simulink model "atrias_system_testing_delay"  (R2014a)
settings: Solver=FixedStepDiscrete  StartTime=0.0  StopTime=inf  FixedStep=sample_time  RelTol=1e-3
PreLoadFcn:
  | set_sampletime
PostLoadFcn:
  | set_sampletime
InitFcn:
  | sys_params
StartFcn:
  | set_sampletime
values from neighbouring files (symbols this model uses):
  A_lpf_velocity = 1 + B1_lpf_velocity + B2_lpf_velocity    [daq_params_osu.m]
  B1_lpf_velocity = -2*exp(-lpf_damping*fcut_velocity*sample_time)*cos(fcut_velocity*sample_time*sqrt(1-lpf_damping^2))    [daq_params_osu.m]
  B2_lpf_velocity = exp(-2*lpf_damping*fcut_velocity*sample_time)    [daq_params_osu.m]
  BOOM_MAX_ENCODER_TICKS = 2^17 - 1    (= 131071)    [daq_params_osu.m]
  BOOM_PITCH_CAL_VALUE_RAD = 0    [daq_params_osu.m]
  BOOM_PITCH_CAL_VALUE_TICKS = 43809    [daq_params_osu.m]
  BOOM_PITCH_ENCODER_RAD_PER_TICK = -2*pi / (2^17 * 2)    (= -2.39684498107e-05)    [daq_params_osu.m]
  BOOM_ROLL_CAL_VALUE_RAD = 0.1271    [daq_params_osu.m]
  BOOM_ROLL_CAL_VALUE_TICKS = 9318    [daq_params_osu.m]
  BOOM_ROLL_ENCODER_RAD_PER_TICK = 2*pi / (2^17 * 7)    (= 6.84812851735e-06)    [daq_params_osu.m]
  BOOM_YAW_ENCODER_RAD_PER_TICK = 2*pi / (2^17 * 9.6)    (= 4.9934270439e-06)    [daq_params_osu.m]
  CURRENT_LIMIT = 100    [daq_params_osu.m]
  fcut_smooth = 16*(2*pi)    (= 100.530964915)    [daq_params_osu.m]
  fcut_unwrap = 8*(2*pi)    (= 50.2654824574)    [daq_params_osu.m]
  gui_disable_cmd = 0    [daq_params_osu.m]
  gui_enable_cmd = 0    [daq_params_osu.m]
  gui_estop_cmd = 0    [daq_params_osu.m]
  gui_reset_cmd = 0    [daq_params_osu.m]
  HIP_ABS_ENCODER_RAD_PER_TICK = 2*pi / 2^13    (= 0.000766990393943)    [daq_params_osu.m]
  HIP_ABS_MAX_ENCODER_TICKS = 2^13 - 1    (= 8191)    [daq_params_osu.m]
  HIP_INC_ENCODER_RAD_PER_TICK = 2*pi / (2500 * 4 * 57)    (= 1.10231321179e-05)    [daq_params_osu.m]
  HIP_INC_MAX_ENCODER_TICKS = 2^16 - 1    (= 65535)    [daq_params_osu.m]
  HIP_MOTOR_CONSTANT = 0.184    [daq_params_osu.m]
  HIP_MTR_GEAR_RATIO = 57    [daq_params_osu.m]
  HIP_MTR_MAX_TORQUE = MTR_HIP_MAX_CURRENT*HIP_MOTOR_CONSTANT*HIP_MTR_GEAR_RATIO    (= 629.28)    [daq_params_osu.m]
  INC_ENC_DIRS = -[ LEG1_MOTOR_A_DIRECTION ... (first row only)    [daq_params_osu.m]
  INC_ENC_RAD_PER_TICK = 2*pi/14000/LEG_MTR_GEAR_RATIO    (= 8.97597901026e-06)    [daq_params_osu.m]
  k_sea = 4118    [sys_params.m]
  LEFT_HIP_CALIB_POS = 0    [daq_params_osu.m]
  LEFT_HIP_CALIB_VAL = 7192 - 2^13    (= -1000)    [daq_params_osu.m]
  LEFT_MOTOR_HIP_DIRECTION = -1.0    (= -1)    [daq_params_osu.m]
  LEG1_LEG_A_CALIB_VAL = 265417675    [daq_params_osu.m]
  LEG1_LEG_A_RAD_PER_CNT = -9.8039216e-09    [daq_params_osu.m]
  LEG1_LEG_B_CALIB_VAL = 175319150    [daq_params_osu.m]
  LEG1_LEG_B_RAD_PER_CNT = -9.8039216e-09    [daq_params_osu.m]
  LEG1_MOTOR_A_DIRECTION = -1.0    (= -1)    [daq_params_osu.m]
  LEG1_MOTOR_B_DIRECTION = -1.0    (= -1)    [daq_params_osu.m]
  LEG1_TRAN_A_CALIB_VAL = 143046540    [daq_params_osu.m]
  LEG1_TRAN_A_RAD_PER_CNT = 9.8039216e-09    [daq_params_osu.m]
  LEG1_TRAN_B_CALIB_VAL = 142356572    [daq_params_osu.m]
  LEG1_TRAN_B_RAD_PER_CNT = -9.8039216e-09    [daq_params_osu.m]
  LEG2_LEG_A_CALIB_VAL = 264357825    [daq_params_osu.m]
  LEG2_LEG_A_RAD_PER_CNT = -9.8039216e-09    [daq_params_osu.m]
  LEG2_LEG_B_CALIB_VAL = 261444054    [daq_params_osu.m]
  LEG2_LEG_B_RAD_PER_CNT = 9.8039216e-09    [daq_params_osu.m]
  LEG2_MOTOR_A_DIRECTION = 1.0    (= 1)    [daq_params_osu.m]
  LEG2_MOTOR_B_DIRECTION = 1.0    (= 1)    [daq_params_osu.m]
  LEG2_TRAN_A_CALIB_VAL = 142300933    [daq_params_osu.m]
  LEG2_TRAN_A_RAD_PER_CNT = 9.8039216e-09    [daq_params_osu.m]
  LEG2_TRAN_B_CALIB_VAL = 142287413    [daq_params_osu.m]
  LEG2_TRAN_B_RAD_PER_CNT = -9.8039216e-09    [daq_params_osu.m]
  LEG_A_CALIB_LOC = pi + 0.305432619099008    (= 3.44702527269)    [daq_params_osu.m]
  LEG_B_CALIB_LOC = pi - 0.305432619099008    (= 2.83616003449)    [daq_params_osu.m]
  LEG_MOTOR_CONSTANT = 0.119    [daq_params_osu.m]
  LEG_MTR_GEAR_RATIO = 50    [daq_params_osu.m]
  LEG_MTR_MAX_TORQUE = MTR_MAX_CURRENT*LEG_MOTOR_CONSTANT*LEG_MTR_GEAR_RATIO    (= 922.25)    [daq_params_osu.m]
  max_encoder_velocity = 200    [daq_params_osu.m]
  MEDULLA_ADC_MAX_VOLTS = 2.70    (= 2.7)    [daq_params_osu.m]
  MEDULLA_ADC_OFFSET_COUNTS = 172    [daq_params_osu.m]
  MEDULLA_STATE_ERROR = 5    [daq_params_osu.m]
  MEDULLA_STATE_HALT = 4    [daq_params_osu.m]
  MEDULLA_STATE_IDLE = 0    [daq_params_osu.m]
  MEDULLA_STATE_RESET = 6    [daq_params_osu.m]
  MEDULLA_STATE_RUN = 2    [daq_params_osu.m]
  MEDULLA_TIMER_FREQ = 32e6    (= 32000000)    [daq_params_osu.m]
  MOTOR_POSITION_LIMITS_LOWER = [2.5; 1.4; 0.4]    [daq_params_osu.m]
  MOTOR_POSITION_LIMITS_UPPER = [4.9; 3.8; 2.5]    [daq_params_osu.m]
  MTR_HIP_MAX_CURRENT = 60.0    (= 60)    [daq_params_osu.m]
  MTR_MAX_CONT_CURRENT = 100.0    (= 100)    [daq_params_osu.m]
  MTR_MAX_COUNT = 19900    [daq_params_osu.m]
  MTR_MAX_CURRENT = 155.0    (= 155)    [daq_params_osu.m]
  nom_sample_time = 0.001    [sys_params.m]
  RIGHT_HIP_CALIB_POS = 0    [daq_params_osu.m]
  RIGHT_HIP_CALIB_VAL = 1091    [daq_params_osu.m]
  RIGHT_MOTOR_HIP_DIRECTION = 1.0    (= 1)    [daq_params_osu.m]
  sample_time = 1/update_freq    (= 0.001)    [daq_params_osu.m]
  sensor_start_time = 8    [daq_params_osu.m]
undefined symbols (not defined in the file or in its folder): max_sensor_velocity
libraries: xpcethercatlib x196, simulink x50, slrtlib x4, dspswit3 x1
(part 4 of 4)

== system atrias_system_testing_delay/DAQ/Elmo Back Right/Drive state transition ==
  Status : Inport
  Bitwise Operator : simulink/Logic and Bit Operations/Bitwise Operator  logicop=AND  UseBitMask=on  BitMask=hex2dec('ff')  BitMaskRealWorld=Stored Integer
  Bitwise Operator1 : simulink/Logic and Bit Operations/Bitwise Operator  logicop=AND  UseBitMask=on  BitMask=hex2dec('80')  BitMaskRealWorld=Stored Integer
  Compare To Constant : simulink/Logic and Bit Operations/Compare To Constant  relop===  const=80  OutDataTypeStr=boolean
  Compare To Constant1 : simulink/Logic and Bit Operations/Compare To Constant  relop===  const=49  OutDataTypeStr=boolean
  Compare To Constant2 : simulink/Logic and Bit Operations/Compare To Constant  relop===  const=51  OutDataTypeStr=boolean
  Compare To Constant3 : simulink/Logic and Bit Operations/Compare To Constant  relop===  const=55  OutDataTypeStr=boolean
  Compare To Zero : simulink/Logic and Bit Operations/Compare To Zero  relop=~=  OutDataTypeStr=boolean
  Constant : Constant  Value=0  OutDataTypeStr=uint16
  Constant1 : Constant  Value=128  OutDataTypeStr=uint16
  Constant2 : Constant  Value=6  OutDataTypeStr=uint16
  Constant3 : Constant  Value=7  OutDataTypeStr=uint16
  Constant4 : Constant  Value=15  OutDataTypeStr=uint16
  Constant5 : Constant  Value=15  OutDataTypeStr=uint16
  Switch{,1..4} (5 alike) : Switch  Criteria=u2 > Threshold
  Control : Outport
  wires:
  Status/1 -> Bitwise Operator/1, Bitwise Operator1/1
  Bitwise Operator1/1 -> Compare To Zero/1
  Compare To Zero/1 -> Switch/2
  Constant1/1 -> Switch/1
  Constant/1 -> Switch/3
  Compare To Constant/1 -> Switch1/2
  Switch/1 -> Switch1/3
  Bitwise Operator/1 -> Compare To Constant3/1, Compare To Constant2/1, Compare To Constant1/1, Compare To Constant/1
  Constant2/1 -> Switch1/1
  Compare To Constant1/1 -> Switch2/2
  Switch1/1 -> Switch2/3
  Constant3/1 -> Switch2/1
  Compare To Constant2/1 -> Switch3/2
  Switch2/1 -> Switch3/3
  Constant4/1 -> Switch3/1
  Compare To Constant3/1 -> Switch4/2
  Switch3/1 -> Switch4/3
  Constant5/1 -> Switch4/1
  Switch4/1 -> Control/1

== system atrias_system_testing_delay/DAQ/Elmo Front Left/Drive state transition ==
  Status : Inport
  Bitwise Operator : simulink/Logic and Bit Operations/Bitwise Operator  logicop=AND  UseBitMask=on  BitMask=hex2dec('ff')  BitMaskRealWorld=Stored Integer
  Bitwise Operator1 : simulink/Logic and Bit Operations/Bitwise Operator  logicop=AND  UseBitMask=on  BitMask=hex2dec('80')  BitMaskRealWorld=Stored Integer
  Compare To Constant : simulink/Logic and Bit Operations/Compare To Constant  relop===  const=80  OutDataTypeStr=boolean
  Compare To Constant1 : simulink/Logic and Bit Operations/Compare To Constant  relop===  const=49  OutDataTypeStr=boolean
  Compare To Constant2 : simulink/Logic and Bit Operations/Compare To Constant  relop===  const=51  OutDataTypeStr=boolean
  Compare To Constant3 : simulink/Logic and Bit Operations/Compare To Constant  relop===  const=55  OutDataTypeStr=boolean
  Compare To Zero : simulink/Logic and Bit Operations/Compare To Zero  relop=~=  OutDataTypeStr=boolean
  Constant : Constant  Value=0  OutDataTypeStr=uint16
  Constant1 : Constant  Value=128  OutDataTypeStr=uint16
  Constant2 : Constant  Value=6  OutDataTypeStr=uint16
  Constant3 : Constant  Value=7  OutDataTypeStr=uint16
  Constant4 : Constant  Value=15  OutDataTypeStr=uint16
  Constant5 : Constant  Value=15  OutDataTypeStr=uint16
  Switch{,1..4} (5 alike) : Switch  Criteria=u2 > Threshold
  Control : Outport
  wires:
  Status/1 -> Bitwise Operator/1, Bitwise Operator1/1
  Bitwise Operator1/1 -> Compare To Zero/1
  Compare To Zero/1 -> Switch/2
  Constant1/1 -> Switch/1
  Constant/1 -> Switch/3
  Compare To Constant/1 -> Switch1/2
  Switch/1 -> Switch1/3
  Bitwise Operator/1 -> Compare To Constant3/1, Compare To Constant2/1, Compare To Constant1/1, Compare To Constant/1
  Constant2/1 -> Switch1/1
  Compare To Constant1/1 -> Switch2/2
  Switch1/1 -> Switch2/3
  Constant3/1 -> Switch2/1
  Compare To Constant2/1 -> Switch3/2
  Switch2/1 -> Switch3/3
  Constant4/1 -> Switch3/1
  Compare To Constant3/1 -> Switch4/2
  Switch3/1 -> Switch4/3
  Constant5/1 -> Switch4/1
  Switch4/1 -> Control/1

== system atrias_system_testing_delay/DAQ/Elmo Front Right/Drive state transition ==
  Status : Inport
  Bitwise Operator : simulink/Logic and Bit Operations/Bitwise Operator  logicop=AND  UseBitMask=on  BitMask=hex2dec('ff')  BitMaskRealWorld=Stored Integer
  Bitwise Operator1 : simulink/Logic and Bit Operations/Bitwise Operator  logicop=AND  UseBitMask=on  BitMask=hex2dec('80')  BitMaskRealWorld=Stored Integer
  Compare To Constant : simulink/Logic and Bit Operations/Compare To Constant  relop===  const=80  OutDataTypeStr=boolean
  Compare To Constant1 : simulink/Logic and Bit Operations/Compare To Constant  relop===  const=49  OutDataTypeStr=boolean
  Compare To Constant2 : simulink/Logic and Bit Operations/Compare To Constant  relop===  const=51  OutDataTypeStr=boolean
  Compare To Constant3 : simulink/Logic and Bit Operations/Compare To Constant  relop===  const=55  OutDataTypeStr=boolean
  Compare To Zero : simulink/Logic and Bit Operations/Compare To Zero  relop=~=  OutDataTypeStr=boolean
  Constant : Constant  Value=0  OutDataTypeStr=uint16
  Constant1 : Constant  Value=128  OutDataTypeStr=uint16
  Constant2 : Constant  Value=6  OutDataTypeStr=uint16
  Constant3 : Constant  Value=7  OutDataTypeStr=uint16
  Constant4 : Constant  Value=15  OutDataTypeStr=uint16
  Constant5 : Constant  Value=15  OutDataTypeStr=uint16
  Switch{,1..4} (5 alike) : Switch  Criteria=u2 > Threshold
  Control : Outport
  wires:
  Status/1 -> Bitwise Operator/1, Bitwise Operator1/1
  Bitwise Operator1/1 -> Compare To Zero/1
  Compare To Zero/1 -> Switch/2
  Constant1/1 -> Switch/1
  Constant/1 -> Switch/3
  Compare To Constant/1 -> Switch1/2
  Switch/1 -> Switch1/3
  Bitwise Operator/1 -> Compare To Constant3/1, Compare To Constant2/1, Compare To Constant1/1, Compare To Constant/1
  Constant2/1 -> Switch1/1
  Compare To Constant1/1 -> Switch2/2
  Switch1/1 -> Switch2/3
  Constant3/1 -> Switch2/1
  Compare To Constant2/1 -> Switch3/2
  Switch2/1 -> Switch3/3
  Constant4/1 -> Switch3/1
  Compare To Constant3/1 -> Switch4/2
  Switch3/1 -> Switch4/3
  Constant5/1 -> Switch4/1
  Switch4/1 -> Control/1

== system atrias_system_testing_delay/DAQ/calibrate_and_convert_to_rad/calibrate_abs_encoder ==
  encoder_ticks : Inport
  cal_pt_ticks : Inport  Port=2
  cal_pt_rad : Inport  Port=3
  ticks_to_rad_const : Inport  Port=4
  Product : Product  RndMeth=Zero
  Sum : Sum  Inputs=|+-
  Sum1 : Sum  Inputs=|++
  angle [rad] : Outport
  wires:
  Sum/1 -> Product/1  "tick_diff"
  encoder_ticks/1 -> Sum/1  "encoder_ticks"
  Product/1 -> Sum1/1  "rad_diff"
  ticks_to_rad_const/1 -> Product/2  "ticks_to_rad_const"
  cal_pt_ticks/1 -> Sum/2  "calibration_point_ticks"
  Sum1/1 -> angle [rad]/1  "calibrated_angle"
  cal_pt_rad/1 -> Sum1/2  "calibration_point_radians"

== system atrias_system_testing_delay/DAQ/calibrate_and_convert_to_rad/calibration_pt_radians ==
  Constant{1,3,5,7} (4 alike) : Constant  Value=LEG_A_CALIB_LOC
  Constant10 : Constant  Value=RIGHT_HIP_CALIB_POS
  Constant11 : Constant  Value=BOOM_ROLL_CAL_VALUE_RAD
  Constant12 : Constant  Value=BOOM_PITCH_CAL_VALUE_RAD
  Constant{2,4,6,8} (4 alike) : Constant  Value=LEG_B_CALIB_LOC
  Constant9 : Constant  Value=LEFT_HIP_CALIB_POS
  Mux3 : Mux  Inputs=12
  calibration_pt [rad] : Outport
  wires:
  Constant4/1 -> Mux3/4
  Constant8/1 -> Mux3/8
  Constant3/1 -> Mux3/1
  Mux3/1 -> calibration_pt [rad]/1
  Constant11/1 -> Mux3/11
  Constant6/1 -> Mux3/7
  Constant12/1 -> Mux3/12
  Constant9/1 -> Mux3/10
  Constant2/1 -> Mux3/3
  Constant5/1 -> Mux3/6
  Constant1/1 -> Mux3/2
  Constant10/1 -> Mux3/9
  Constant7/1 -> Mux3/5

== system atrias_system_testing_delay/DAQ/calibrate_and_convert_to_rad/calibration_pt_ticks ==
  Constant1 : Constant  Value=LEG2_TRAN_A_CALIB_VAL
  Constant10 : Constant  Value=RIGHT_HIP_CALIB_VAL
  Constant11 : Constant  Value=BOOM_ROLL_CAL_VALUE_TICKS
  Constant12 : Constant  Value=BOOM_PITCH_CAL_VALUE_TICKS
  Constant2 : Constant  Value=LEG2_LEG_B_CALIB_VAL
  Constant3 : Constant  Value=LEG2_LEG_A_CALIB_VAL
  Constant4 : Constant  Value=LEG2_TRAN_B_CALIB_VAL
  Constant5 : Constant  Value=LEG1_TRAN_A_CALIB_VAL
  Constant6 : Constant  Value=LEG1_LEG_B_CALIB_VAL
  Constant7 : Constant  Value=LEG1_LEG_A_CALIB_VAL
  Constant8 : Constant  Value=LEG1_TRAN_B_CALIB_VAL
  Constant9 : Constant  Value=LEFT_HIP_CALIB_VAL
  Mux3 : Mux  Inputs=12
  calibration_pt [ticks] : Outport
  wires:
  Constant3/1 -> Mux3/5
  Constant10/1 -> Mux3/9
  Constant5/1 -> Mux3/2
  Constant1/1 -> Mux3/6
  Constant6/1 -> Mux3/3
  Constant9/1 -> Mux3/10
  Constant12/1 -> Mux3/12
  Constant2/1 -> Mux3/7
  Constant11/1 -> Mux3/11
  Mux3/1 -> calibration_pt [ticks]/1
  Constant7/1 -> Mux3/1
  Constant4/1 -> Mux3/8
  Constant8/1 -> Mux3/4

== system atrias_system_testing_delay/DAQ/calibrate_and_convert_to_rad/ticks_to_radians_constants ==
  Constant1 : Constant  Value=LEG2_TRAN_A_RAD_PER_CNT
  Constant10 : Constant  Value=-HIP_ABS_ENCODER_RAD_PER_TICK
  Constant11 : Constant  Value=BOOM_ROLL_ENCODER_RAD_PER_TICK
  Constant12 : Constant  Value=BOOM_PITCH_ENCODER_RAD_PER_TICK
  Constant2 : Constant  Value=LEG2_LEG_B_RAD_PER_CNT
  Constant3 : Constant  Value=LEG2_LEG_A_RAD_PER_CNT
  Constant4 : Constant  Value=LEG2_TRAN_B_RAD_PER_CNT
  Constant5 : Constant  Value=LEG1_TRAN_A_RAD_PER_CNT
  Constant6 : Constant  Value=LEG1_LEG_B_RAD_PER_CNT
  Constant7 : Constant  Value=LEG1_LEG_A_RAD_PER_CNT
  Constant8 : Constant  Value=LEG1_TRAN_B_RAD_PER_CNT
  Constant9 : Constant  Value=HIP_ABS_ENCODER_RAD_PER_TICK
  Mux3 : Mux  Inputs=12
  ticks_to_rad_constants : Outport
  wires:
  Constant3/1 -> Mux3/5
  Constant9/1 -> Mux3/9
  Constant5/1 -> Mux3/2
  Constant1/1 -> Mux3/6
  Constant6/1 -> Mux3/3
  Constant10/1 -> Mux3/10
  Constant12/1 -> Mux3/12
  Constant2/1 -> Mux3/7
  Constant11/1 -> Mux3/11
  Mux3/1 -> ticks_to_rad_constants/1
  Constant7/1 -> Mux3/1
  Constant4/1 -> Mux3/8
  Constant8/1 -> Mux3/4

== system atrias_system_testing_delay/DAQ/remove_encoder_dropouts/check_error ==
  error : Inport
  Enable : EnablePort
  Compare To Constant : simulink/Logic and Bit Operations/Compare To Constant  relop=<=  const=max_encoder_velocity*sample_time  OutDataTypeStr=boolean
  acceptable? : Outport  InitialOutput=1
  wires:
  error/1 -> Compare To Constant/1
  Compare To Constant/1 -> acceptable?/1

== system atrias_system_testing_delay/DAQ/unwrap_encoders/unwrap_boom_yaw_encoder ==
  note: Recommended if-then structure for assigning
      | constants. The criterion '~=0' is realized as cpu register
      | shift when compiling.  The resulting code is fast.
  note: Transform Wrapped Angle into Continuous Angle
  note: predicted angle:
      | phi' = phi_(n-1) + dphi
      | = phi_(n-1) + phi_(n-1)-phi_(n-2)
  wrapped [ticks] : Inport
  1/BOOM_MAX_ENCODER_TICKS : Gain  Gain=1/BOOM_MAX_ENCODER_TICKS
  Abs : Abs
  BOOM_MAX_ENCODER_TICKS : Gain  Gain=BOOM_MAX_ENCODER_TICKS
  Compare To Zero : simulink/Logic and Bit Operations/Compare To Zero  relop=>  OutDataTypeStr=uint8
  Discrete Single Pole Lowpass Filter : DiscreteTransferFcn  Numerator=[(1-exp(-2*pi*fcut_unwrap*sample_time)) 0]  Denominator=[1 -exp(-2*pi*fcut_unwrap*sample_time)]  SampleTime=sample_time
  Gain2 : Gain  Gain=2
  Product : Product  RndMeth=Zero
  Rounding Function : Rounding
  Sum : Sum  Inputs=|+-
  Sum1 : Sum  Inputs=|++
  Sum2 : Sum  Inputs=|++
  Sum3 : Sum  Inputs=-+|
  Switch : Switch  Criteria=u2 ~= 0
      settings: AttributesFormatString=%<Criteria>
  Unit Delay phi_(n-1) : UnitDelay  SampleTime=-1
      settings: AttributesFormatString=initial condition = %<X0>
  Unit Delay phi_(n-2) : UnitDelay  SampleTime=-1
      settings: AttributesFormatString=initial condition = %<X0>
  const : Constant  Value=0.5
  no : Constant  Value=-1
  yes : Constant
  continuous [ticks] : Outport
  wires:
  Discrete Single Pole Lowpass Filter/1 -> Unit Delay phi_(n-1)/1
  Compare To Zero/1 -> Switch/2
  Unit Delay phi_(n-2)/1 -> Sum/2
  yes/1 -> Switch/1
  no/1 -> Switch/3
  Switch/1 -> Product/2
  Rounding Function/1 -> BOOM_MAX_ENCODER_TICKS/1
  wrapped [ticks]/1 -> Sum1/1, Sum3/1
  Product/1 -> Sum1/2
  Abs/1 -> 1/BOOM_MAX_ENCODER_TICKS/1
  1/BOOM_MAX_ENCODER_TICKS/1 -> Sum2/1
  const/1 -> Sum2/2
  Sum2/1 -> Rounding Function/1
  Sum1/1 -> continuous [ticks]/1, Discrete Single Pole Lowpass Filter/1
  BOOM_MAX_ENCODER_TICKS/1 -> Product/1
  Unit Delay phi_(n-1)/1 -> Unit Delay phi_(n-2)/1, Gain2/1
  Gain2/1 -> Sum/1
  Sum/1 -> Sum3/2
  Sum3/1 -> Abs/1, Compare To Zero/1  "phi'-phi"

== system atrias_system_testing_delay/DAQ/unwrap_encoders/unwrap_lateral_absolute_encoders Left ==
  note: predicted angle:
      | phi' = phi_(n-1) + dphi
      | = phi_(n-1) + phi_(n-1)-phi_(n-2)
  note: Transform Wrapped Angle into Continuous Angle
  note: Recommended if-then structure for assigning
      | constants. The criterion '~=0' is realized as cpu register
      | shift when compiling.  The resulting code is fast.
  wrapped [ticks] : Inport
  1/HIP_ABS_MAX_ENCODER_TICKS : Gain  Gain=1/HIP_ABS_MAX_ENCODER_TICKS
  Abs : Abs
  Compare To Zero : simulink/Logic and Bit Operations/Compare To Zero  relop=>  OutDataTypeStr=uint8
  Discrete Single Pole Lowpass Filter : DiscreteTransferFcn  Numerator=[(1-exp(-2*pi*fcut_unwrap*sample_time)) 0]  Denominator=[1 -exp(-2*pi*fcut_unwrap*sample_time)]  SampleTime=sample_time
  Gain2 : Gain  Gain=2
  HIP_ABS_MAX_ENCODER_TICKS : Gain  Gain=HIP_ABS_MAX_ENCODER_TICKS
  Product : Product  RndMeth=Zero
  Rounding Function : Rounding
  Sum : Sum  Inputs=|+-
  Sum1 : Sum  Inputs=|++
  Sum2 : Sum  Inputs=|++
  Sum3 : Sum  Inputs=-+|
  Switch : Switch  Criteria=u2 ~= 0
      settings: AttributesFormatString=%<Criteria>
  Unit Delay phi_(n-1) : UnitDelay  SampleTime=-1
      settings: AttributesFormatString=initial condition = %<X0>
  Unit Delay phi_(n-2) : UnitDelay  SampleTime=-1
      settings: AttributesFormatString=initial condition = %<X0>
  const : Constant  Value=0.5
  no : Constant  Value=-1
  yes : Constant
  continuous [ticks] : Outport
  wires:
  Sum3/1 -> Compare To Zero/1, Abs/1  "phi'-phi"
  Sum/1 -> Sum3/2
  Gain2/1 -> Sum/1
  Unit Delay phi_(n-1)/1 -> Gain2/1, Unit Delay phi_(n-2)/1
  HIP_ABS_MAX_ENCODER_TICKS/1 -> Product/1
  Sum1/1 -> continuous [ticks]/1, Discrete Single Pole Lowpass Filter/1
  Sum2/1 -> Rounding Function/1
  const/1 -> Sum2/2
  1/HIP_ABS_MAX_ENCODER_TICKS/1 -> Sum2/1
  Abs/1 -> 1/HIP_ABS_MAX_ENCODER_TICKS/1
  Product/1 -> Sum1/2
  wrapped [ticks]/1 -> Sum3/1, Sum1/1
  Rounding Function/1 -> HIP_ABS_MAX_ENCODER_TICKS/1
  Switch/1 -> Product/2
  no/1 -> Switch/3
  yes/1 -> Switch/1
  Unit Delay phi_(n-2)/1 -> Sum/2
  Compare To Zero/1 -> Switch/2
  Discrete Single Pole Lowpass Filter/1 -> Unit Delay phi_(n-1)/1

== system atrias_system_testing_delay/DAQ/unwrap_encoders/unwrap_lateral_absolute_encoders Right ==
  note: Recommended if-then structure for assigning
      | constants. The criterion '~=0' is realized as cpu register
      | shift when compiling.  The resulting code is fast.
  note: Transform Wrapped Angle into Continuous Angle
  note: predicted angle:
      | phi' = phi_(n-1) + dphi
      | = phi_(n-1) + phi_(n-1)-phi_(n-2)
  wrapped [ticks] : Inport
  1/HIP_ABS_MAX_ENCODER_TICKS : Gain  Gain=1/HIP_ABS_MAX_ENCODER_TICKS
  Abs : Abs
  Compare To Zero : simulink/Logic and Bit Operations/Compare To Zero  relop=>  OutDataTypeStr=uint8
  Discrete Single Pole Lowpass Filter : DiscreteTransferFcn  Numerator=[(1-exp(-2*pi*fcut_unwrap*sample_time)) 0]  Denominator=[1 -exp(-2*pi*fcut_unwrap*sample_time)]  SampleTime=sample_time
  Gain2 : Gain  Gain=2
  HIP_ABS_MAX_ENCODER_TICKS : Gain  Gain=HIP_ABS_MAX_ENCODER_TICKS
  Product : Product  RndMeth=Zero
  Rounding Function : Rounding
  Sum : Sum  Inputs=|+-
  Sum1 : Sum  Inputs=|++
  Sum2 : Sum  Inputs=|++
  Sum3 : Sum  Inputs=-+|
  Switch : Switch  Criteria=u2 ~= 0
      settings: AttributesFormatString=%<Criteria>
  Unit Delay phi_(n-1) : UnitDelay  SampleTime=-1
      settings: AttributesFormatString=initial condition = %<X0>
  Unit Delay phi_(n-2) : UnitDelay  SampleTime=-1
      settings: AttributesFormatString=initial condition = %<X0>
  const : Constant  Value=0.5
  no : Constant  Value=-1
  yes : Constant
  continuous [ticks] : Outport
  wires:
  Discrete Single Pole Lowpass Filter/1 -> Unit Delay phi_(n-1)/1
  Compare To Zero/1 -> Switch/2
  Unit Delay phi_(n-2)/1 -> Sum/2
  yes/1 -> Switch/1
  no/1 -> Switch/3
  Switch/1 -> Product/2
  Rounding Function/1 -> HIP_ABS_MAX_ENCODER_TICKS/1
  wrapped [ticks]/1 -> Sum1/1, Sum3/1
  Product/1 -> Sum1/2
  Abs/1 -> 1/HIP_ABS_MAX_ENCODER_TICKS/1
  1/HIP_ABS_MAX_ENCODER_TICKS/1 -> Sum2/1
  const/1 -> Sum2/2
  Sum2/1 -> Rounding Function/1
  Sum1/1 -> Discrete Single Pole Lowpass Filter/1, continuous [ticks]/1
  HIP_ABS_MAX_ENCODER_TICKS/1 -> Product/1
  Unit Delay phi_(n-1)/1 -> Unit Delay phi_(n-2)/1, Gain2/1
  Gain2/1 -> Sum/1
  Sum/1 -> Sum3/2
  Sum3/1 -> Abs/1, Compare To Zero/1  "phi'-phi"

== system atrias_system_testing_delay/DAQ/unwrap_encoders/unwrap_lateral_incremental_encoders Left ==
  note: Recommended if-then structure for assigning
      | constants. The criterion '~=0' is realized as cpu register
      | shift when compiling.  The resulting code is fast.
  note: Transform Wrapped Angle into Continuous Angle
  note: predicted angle:
      | phi' = phi_(n-1) + dphi
      | = phi_(n-1) + phi_(n-1)-phi_(n-2)
  wrapped [ticks] : Inport
  1/HIP_INC_MAX_ENCODER_TICKS : Gain  Gain=1/HIP_INC_MAX_ENCODER_TICKS
  Abs : Abs
  Compare To Zero : simulink/Logic and Bit Operations/Compare To Zero  relop=>  OutDataTypeStr=uint8
  Discrete Single Pole Lowpass Filter : DiscreteTransferFcn  Numerator=[(1-exp(-2*pi*fcut_unwrap*sample_time)) 0]  Denominator=[1 -exp(-2*pi*fcut_unwrap*sample_time)]  SampleTime=sample_time
  Gain2 : Gain  Gain=2
  HIP_INC_MAX_ENCODER_TICKS : Gain  Gain=HIP_INC_MAX_ENCODER_TICKS
  Product : Product  RndMeth=Zero
  Rounding Function : Rounding
  Sum : Sum  Inputs=|+-
  Sum1 : Sum  Inputs=|++
  Sum2 : Sum  Inputs=|++
  Sum3 : Sum  Inputs=-+|
  Switch : Switch  Criteria=u2 ~= 0
      settings: AttributesFormatString=%<Criteria>
  Unit Delay phi_(n-1) : UnitDelay  SampleTime=-1
      settings: AttributesFormatString=initial condition = %<X0>
  Unit Delay phi_(n-2) : UnitDelay  SampleTime=-1
      settings: AttributesFormatString=initial condition = %<X0>
  const : Constant  Value=0.5
  no : Constant  Value=-1
  yes : Constant
  continuous [ticks] : Outport
  wires:
  Discrete Single Pole Lowpass Filter/1 -> Unit Delay phi_(n-1)/1
  Compare To Zero/1 -> Switch/2
  Unit Delay phi_(n-2)/1 -> Sum/2
  yes/1 -> Switch/1
  no/1 -> Switch/3
  Switch/1 -> Product/2
  Rounding Function/1 -> HIP_INC_MAX_ENCODER_TICKS/1
  wrapped [ticks]/1 -> Sum1/1, Sum3/1
  Product/1 -> Sum1/2
  Abs/1 -> 1/HIP_INC_MAX_ENCODER_TICKS/1
  1/HIP_INC_MAX_ENCODER_TICKS/1 -> Sum2/1
  const/1 -> Sum2/2
  Sum2/1 -> Rounding Function/1
  Sum1/1 -> Discrete Single Pole Lowpass Filter/1, continuous [ticks]/1
  HIP_INC_MAX_ENCODER_TICKS/1 -> Product/1
  Unit Delay phi_(n-1)/1 -> Unit Delay phi_(n-2)/1, Gain2/1
  Gain2/1 -> Sum/1
  Sum/1 -> Sum3/2
  Sum3/1 -> Abs/1, Compare To Zero/1  "phi'-phi"

== system atrias_system_testing_delay/DAQ/unwrap_encoders/unwrap_lateral_incremental_encoders Right ==
  note: predicted angle:
      | phi' = phi_(n-1) + dphi
      | = phi_(n-1) + phi_(n-1)-phi_(n-2)
  note: Transform Wrapped Angle into Continuous Angle
  note: Recommended if-then structure for assigning
      | constants. The criterion '~=0' is realized as cpu register
      | shift when compiling.  The resulting code is fast.
  wrapped [ticks] : Inport
  1/HIP_INC_MAX_ENCODER_TICKS : Gain  Gain=1/HIP_INC_MAX_ENCODER_TICKS
  Abs : Abs
  Compare To Zero : simulink/Logic and Bit Operations/Compare To Zero  relop=>  OutDataTypeStr=uint8
  Discrete Single Pole Lowpass Filter : DiscreteTransferFcn  Numerator=[(1-exp(-2*pi*fcut_unwrap*sample_time)) 0]  Denominator=[1 -exp(-2*pi*fcut_unwrap*sample_time)]  SampleTime=sample_time
  Gain2 : Gain  Gain=2
  HIP_INC_MAX_ENCODER_TICKS : Gain  Gain=HIP_INC_MAX_ENCODER_TICKS
  Product : Product  RndMeth=Zero
  Rounding Function : Rounding
  Sum : Sum  Inputs=|+-
  Sum1 : Sum  Inputs=|++
  Sum2 : Sum  Inputs=|++
  Sum3 : Sum  Inputs=-+|
  Switch : Switch  Criteria=u2 ~= 0
      settings: AttributesFormatString=%<Criteria>
  Unit Delay phi_(n-1) : UnitDelay  SampleTime=-1
      settings: AttributesFormatString=initial condition = %<X0>
  Unit Delay phi_(n-2) : UnitDelay  SampleTime=-1
      settings: AttributesFormatString=initial condition = %<X0>
  const : Constant  Value=0.5
  no : Constant  Value=-1
  yes : Constant
  continuous [ticks] : Outport
  wires:
  Sum3/1 -> Compare To Zero/1, Abs/1  "phi'-phi"
  Sum/1 -> Sum3/2
  Gain2/1 -> Sum/1
  Unit Delay phi_(n-1)/1 -> Gain2/1, Unit Delay phi_(n-2)/1
  HIP_INC_MAX_ENCODER_TICKS/1 -> Product/1
  Sum1/1 -> continuous [ticks]/1, Discrete Single Pole Lowpass Filter/1
  Sum2/1 -> Rounding Function/1
  const/1 -> Sum2/2
  1/HIP_INC_MAX_ENCODER_TICKS/1 -> Sum2/1
  Abs/1 -> 1/HIP_INC_MAX_ENCODER_TICKS/1
  Product/1 -> Sum1/2
  wrapped [ticks]/1 -> Sum3/1, Sum1/1
  Rounding Function/1 -> HIP_INC_MAX_ENCODER_TICKS/1
  Switch/1 -> Product/2
  no/1 -> Switch/3
  yes/1 -> Switch/1
  Unit Delay phi_(n-2)/1 -> Sum/2
  Compare To Zero/1 -> Switch/2
  Discrete Single Pole Lowpass Filter/1 -> Unit Delay phi_(n-1)/1

== matlab function atrias_system_testing_delay/DAQ/logic_voltage_volts ==
  data: u input; volt output; MEDULLA_ADC_OFFSET_COUNTS parameter; MEDULLA_ADC_MAX_VOLTS parameter
function volt = fcn(u, MEDULLA_ADC_OFFSET_COUNTS, MEDULLA_ADC_MAX_VOLTS)
% Taken from Medulla.cpp in the ATRIAS medulla drivers
% at code.google.com/p/atrias
adcReadingVolts = (u - MEDULLA_ADC_OFFSET_COUNTS) * MEDULLA_ADC_MAX_VOLTS/4095;
volt            = 6 * adcReadingVolts;

== matlab function atrias_system_testing_delay/DAQ/medulla_errors ==
  data: u input; errors output
function errors = fcn(u)
% right back, right front, left back, left front, left lateral, right lateral, boom
errors = reshape(bsxfun(@bitand,u,2.^[0 1 2 3 4 5 6 7]),[],1);

== matlab function atrias_system_testing_delay/Compute Medulla State Command ==
  data: medulla_states input uint8; state_cmd output uint8; should_estop input boolean; should_halt input boolean; gui_enable_cmd parameter boolean; gui_disable_cmd parameter boolean; gui_reset_cmd parameter boolean; gui_estop_cmd parameter boolean; MEDULLA_STATE_IDLE parameter uint8; MEDULLA_STATE_RUN parameter uint8; MEDULLA_STATE_HALT parameter uint8; MEDULLA_STATE_ERROR parameter uint8; MEDULLA_STATE_RESET parameter uint8; any_halt output boolean
function [state_cmd,any_halt] = fcn(medulla_states,      ...
                                    should_estop,        ...
                                    should_halt,         ...
                                    gui_enable_cmd,      ...
                                    gui_disable_cmd,     ...
                                    gui_reset_cmd,       ...
                                    gui_estop_cmd,       ...
                                    MEDULLA_STATE_IDLE,  ...
                                    MEDULLA_STATE_RUN,   ...
                                    MEDULLA_STATE_HALT,  ...
                                    MEDULLA_STATE_ERROR, ...
                                    MEDULLA_STATE_RESET)
%#codegen

% Count the number of medullas in each state
any_idle  = any(medulla_states == MEDULLA_STATE_IDLE );
any_reset = any(medulla_states == MEDULLA_STATE_RESET);
any_run   = any(medulla_states == MEDULLA_STATE_RUN  );
any_halt  = any(medulla_states == MEDULLA_STATE_HALT );
any_estop = any(medulla_states == MEDULLA_STATE_ERROR);

% The GUI estop command should do the same thing as asserting the
% should_estop line
should_estop = should_estop || gui_estop_cmd;

% Compute whether or not to reset based on the current states and the
% GUI's input
should_reset = gui_reset_cmd  && ...
              ~gui_enable_cmd && ... % Make sure we're not about to re-enable (precaution)
               any_estop      && ... % A medulla must be e-stopped (precaution)
              ~any_halt       && ... % No medullas may be halting (precaution)
              ~any_run;              % No medullas may be running (precaution)

% Send an E-Stop first if the safeties are engaging, so this can't fail.
% Also send an E-Stop if any medullas are E-stopped, unless the GUI is
% sending a reset command
if ((any_run || any_halt) && should_estop) || (any_estop && ~should_reset)
    state_cmd = MEDULLA_STATE_ERROR;
    return
end

% If any Medullas are halting, automatically command halt for all.
% This is done second as a safety precaution
if any_halt || (any_run && should_halt)
    state_cmd = MEDULLA_STATE_HALT;
    return
end

% Allow for GUI-commanded resets. Make sure an enable command isn't being
% sent as an enable precaution
if should_reset || any_reset
    state_cmd = MEDULLA_STATE_RESET;
    return
end

% Past this point, the robot should be either enabled or disabled
% (no E-Stops or halts)

% Allow the GUI to disable the robot.
% For now, there is no soft shutdown.
if gui_disable_cmd
    state_cmd = MEDULLA_STATE_IDLE;
    return
end

% Allow for enabling (when safeties aren't triggered)
if gui_enable_cmd && ~should_estop && ~should_halt
    state_cmd = MEDULLA_STATE_RUN;
    return
end

% Since we have no errors or relevant GUI commands, just mimic the
% Medullas's current states
if any_idle
    state_cmd = MEDULLA_STATE_IDLE;
    return
else
    state_cmd = MEDULLA_STATE_RUN;
    return
end
end

== matlab function atrias_system_testing_delay/DAQ/motor_temperatures ==
  data: u input; temp output
function temp = fcn(u)
adc_values = ((u - 172.0) * (2.70/(4095.0)));
temp = ((1.0./( (1.0/298.15) + (1.0/3988.0)*log(4700.0./((3.26./adc_values) - 1.0)/10000))) - 273.15);

== matlab function atrias_system_testing_delay/DAQ/motor_voltage_volts ==
  data: u input; volt output
function volt = fcn(u)
volt = (u - 1300.0) * 60.2 / (3600.0 - 1300.0);

== matlab function atrias_system_testing_delay/Update Diagnostics ==
  data: reset input boolean; diags input boolean; diags_out output uint8
function diags_out = fcn(reset, diags)
%#codegen

% Recall the values of our diagnostics through a persistent variable.
% We are using a persistent variable to allow the vector to be resized
% automatically to fit the size of diags
persistent latchedDiags

% Initialize latchedDiags
if isempty(latchedDiags)
    latchedDiags = uint8(zeros(numel(diags), 1));
end


% If we're idle, then reset the counter and forward the diagnostics
% directly through.
if reset
    latchedDiags = uint8(diags);
    diags_out    = uint8(diags);
    return
end

% Since we're not idle, Sequence the diagnostics and latch the
% results    
updates    = diags & (~logical(latchedDiags));
newCounter = max(latchedDiags);
% Protect against counter overflow
if newCounter + 1 > newCounter
    newCounter = newCounter + 1;
end

% Perform the update of newly-activated diagnostic events
latchedDiags(updates) = newCounter;
diags_out             = latchedDiags;

== matlab function atrias_system_testing_delay/DAQ/Limit Switches to Bool ==
  data: sw input; sw_out output boolean
function sw_out  = fcn(sw)
%#codegen

% Binary decode (split the input into an array of booleans)
% This creates a matrix; each column corresponds with one of the original
% input uint8's, and each row corresponds with a bit location within the
% octet.
sw = bsxfun(@bitand, uint8(2.^(0:7)), uint8(sw(2:2:end)))';

% Reshape and cast our output to make Simulink happy
sw_out = logical(sw(:));

== matlab function atrias_system_testing_delay/Mux Diags ==
  data: Halting input; diags output boolean; SW input; ErrorFlags input uint8; ControllerFault input boolean
function diags = fcn(Halting, SW, ErrorFlags, ControllerFault)
%#codegen

% Convert error flags into a boolean array.
% This will generate one column per medulla and one row per bit,
% so when we read it into diags later on it will come out in the right
% order.
ErrorFlags = logical(bsxfun(@bitand, uint8(2.^(0:7)), ErrorFlags))';

% Generate diags from the processed inputs
diags = [ Halting
          SW
          ErrorFlags(:)
          ControllerFault];

== matlab function atrias_system_testing_delay/Demux Diags ==
  data: diags input; halt_diag output; sw1 output; sw2 output; sw3 output; sw4 output; error1 output; error2 output; error3 output; error4 output; error5 output; error6 output; error7 output; contrlr_fault_diag output
function [halt_diag,sw1,sw2,sw3,sw4,error1,error2,error3,error4,error5,error6,error7,contrlr_fault_diag] = fcn(diags)
%#codegen

halt_diag          = diags(1);
sw1                = diags(2:9);
sw2                = diags(10:17);
sw3                = diags(18:25);
sw4                = diags(26:33);
error1             = diags(34:41);
error2             = diags(42:49);
error3             = diags(50:57);
error4             = diags(58:65);
error5             = diags(66:73);
error6             = diags(74:81);
error7             = diags(82:89);
contrlr_fault_diag = diags(90);

== matlab function atrias_system_testing_delay/DAQ/Calc. Rotor Velocities ==
  data: encdiff input; vels_out output double; tsdiff input; cntrdiff input; nom_sample_time parameter; INC_ENC_RAD_PER_TICK parameter; INC_ENC_DIRS parameter; MEDULLA_TIMER_FREQ parameter
function vels_out = fcn(encdiff, tsdiff, cntrdiff, nom_sample_time, INC_ENC_RAD_PER_TICK, INC_ENC_DIRS, MEDULLA_TIMER_FREQ)
%#codegen

% This function calculates the velocities of the motors by differenting the
% positions returned by the rotor encoders. It accounts for varying delta
% times between position samples.
%
% Parameters:
%
%     encdiff   Unwrapped delta between the current and previous encoder value.
%     tsdiff    The difference between the current and previous timestamp value; doesn't need unwrapping!
%     cntrdiff  The (unwrapped) difference between the current and last counter value returned by this medulla (# of cycles since last read).
%
% Returns:
%
%     vels_out  The current rotor velocities (order documented in the Simulink model)


% Current velocity storage; used if we get duplicated data (should a timing issue occur).
% Initialize this to 0 as the robot is probably stopped at master startup.
persistent vels
if isempty(vels)
    vels = zeros(4, 1);
end

% Correct for wraparound
encdiff  = mod(encdiff + 2^15, 2^16) - 2^15;
cntrdiff = mod(cntrdiff, 2^8);

% Decide which values should be updated; we only updated values for which
% we have new data.
updates = logical(cntrdiff);


% Turn an encoder difference (in ticks) into a delta position (in radians).
dpos = double(encdiff) * INC_ENC_RAD_PER_TICK .* INC_ENC_DIRS;

% Compute the delta time between the two subsequent samples. We compensate
% not only for the number of cycles since the last read (cntrdiff) but
% also the difference in relative sensor read times (tsdiff)
dt = nom_sample_time * double(cntrdiff) + tsdiff / MEDULLA_TIMER_FREQ;

% Calculate the velocity using simple finite differencing
newvels = dpos ./ dt;

% Just update those that we have new data for. We "clamp" velocities we
% didn't get data for. This shouldn't be necessary, but is here just in
% case something goes wrong.
vels(updates) = newvels(updates);

% We can't return a persistent variable, so copy the current velocities
% into our return value
vels_out = vels;

== matlab function atrias_system_testing_delay/DAQ/Leg Motor Observer ==
  data: u input double size=[1 6]; q input double; pos output double; rotor_vels input double; vel output; nom_sample_time parameter double; k_sea parameter
function [pos,vel] = fcn(u, q, rotor_vels, nom_sample_time, k_sea)
%#codegen

% Parameters:
%
%     u            Torque commands from the last cycle
%     q            The positional states vector (shouldn't be processed to remove dropouts -- this function does that as well)
%     rotor_vels   The current velocities computed using the incremental encoders in the motors
%     sample_time  The delta time between iterations (parameter defined in daq_params)
%     k_sea        The spring constants for the SEAs (parameter defined in sys_params)
%
% Return values
%
%     pos  A vector of motor positions (order defined below)
%     vel  A vector of motor velocities (order the same as pos)
%
% Order of state, y, etc... (matches rotor velocities):
%     back right
%     front right
%     back left
%     front left
%
% State: first row is position, second is velocity; each column is a
% different motor
%
% Much of the content of this function serves to reject bad absolute
% encoder signals. The 32-bit Renishaw encoders occasionally give bad data
% without setting any error bits. To filter these out, we compare the
% sensed position with the predicted (observed) position. We also look for
% repeated sensed positions, as that occurs when the encoder detects a bad
% reading.
%
% During absolute encoder dropouts, we fill in the missing position data
% using the incremental encoders. Other options for handling dropouts --
% which I have decided against -- include using a second observer design that
% relies only on the incremental encoder (only during dropouts) or just
% trusting the predicted state.


% Set up the system model. We only compute this on startup to save run time.
% Alternatively, we could've directly specified the discrete-time model,
% but I decided it was more readable to specify a continuous-time model and
% transform between the two in code.
persistent A
persistent B

if isempty(A) || isempty(B)
    % Form the continuous-time system model
    inertia = 3.0517; % Reflected moment of inertia (N*m*s^2/rad)
    A_cont  = [0 1; 0 0];
    B_cont  = [0; 1/inertia];
    
    % Translate the continuous-time system model to a discrete one. See
    % Wikipedia for the formula behind this.
    M = [A_cont B_cont; zeros(size(B_cont,2), size(A_cont,2) + size(B_cont,2))];
    M = expm(M * nom_sample_time);
    A = M(1:size(A_cont, 1), 1:size(A_cont, 2));
    B = M(1:size(B_cont, 1), (size(A,2)+1):(size(A,2)+size(B_cont,2)));
end

% Observer gain matrix. Obtained via optimization on existing experimental
% data.
K = [ -0.014305247969510  0.010871733923180
      -7.301581788665865 -0.543374339802686 ];

% Retrieve the measured positions and velocities from the input vectors (in
% the order used by vel, pos, state, ...).
ypos = reshape(q([2 4 6 8]), 1, []);
yvel = reshape(rotor_vels,   1, []);
yleg = reshape(q([1 3 5 7]), 1, []);

% The model (and thus this function) begins running before EtherCAT data is
% available. We need to detect when data becomes available so we don't try
% to observe the state before then.
%
% These state variables are to detect the beginning of data acquisition
% (signaled by ypos changing)
persistent ypos_old
persistent has_data

if isempty(ypos_old) || isempty(has_data)
    ypos_old = ypos;
    has_data = false;
end

% Retain our current state estimate from cycle to cycle (this is the
% observer's memory)
persistent state

% Do initialization for the above state estimate
if isempty(state)
    % This value doesn't really matter; it is ignored while
    % has_data == false and gets reset when has_data becomes true.
    % We do need to get the size right, though, hence the use of ypos and
    % yvel
    state = [ypos; yvel];
end

% Check if we have data yet; if so, send dummy values.
% If we're just initializing now, reset the observer state to the sensed
% state
if ~has_data
    if all(ypos == ypos_old)
        % Not initialized yet; just output dummy data
        pos = pi * ones(1, 4);
        vel = zeros(1, 4);
        return
    else
        % We just got data for the first time! Initialize the observer state
        state    = [ypos; yvel];
        has_data = true;
    end
end

% Determine which position sensors have dropped out. The reasoning for this
% is described above (in the comments at the top of this file).
dropouts = (ypos == ypos_old) | (abs(ypos - state(1,:)) > .2);

% As mentioned above, we fake absolute encoder data during dropouts by
% using the rotor encoders. Assumption: no cycles are missed!
% Missed cycles will cause a drift in ypos for encoders that are currently
% dropped out (and the corresponding motor is moving).
% Assuming no encoders drop out for a long time, this drift will be
% negligible.
ypos(dropouts) = ypos_old(dropouts) + nom_sample_time * yvel(dropouts);

% Update the "old" sensed positions for the next iteration.
ypos_old = ypos;

% Grab the torque commands for the relevant motors (same order as pos, vel,
% state, ...)
u = reshape(u([1 2 4 5]), 1, []);

% Compute the torques generated from the springs. We have no observer for
% the joint angles, so we just trust the sensors there. Since we don't need
% velocities (the damping constant is approximated by zero), the noise is
% negligible.
t_sprngs = k_sea .* (yleg - state(1,:));

% Run the discrete-time observer dynamics (finally!)
state = A * state + B * (u + t_sprngs) + K * (state - [ypos; yvel]);

% Set the function's return values from the current observer state
pos = state(1,:);
vel = state(2,:);

== matlab function atrias_system_testing_delay/Soft limits ==
  data: q input; halt output; dq input; MOTOR_POSITION_LIMITS_UPPER parameter double; MOTOR_POSITION_LIMITS_LOWER parameter double
function halt = fcn(q, ...
                    dq, ...
                    MOTOR_POSITION_LIMITS_UPPER, ...
                    MOTOR_POSITION_LIMITS_LOWER)
%#codegen

ra = q(2) + dq(2) * abs(dq(2)) / (2.0 * 1.7185879 * 30.0);
rb = q(4) + dq(4) * abs(dq(4)) / (2.0 * 1.7185879 * 30.0);
la = q(6) + dq(6) * abs(dq(6)) / (2.0 * 1.7185879 * 30.0);
lb = q(8) + dq(8) * abs(dq(8)) / (2.0 * 1.7185879 * 30.0);
rd = ra - rb;
ld = la - lb;

r = [ra; rb; rd];
l = [la; lb; ld];

halt = any(  r > MOTOR_POSITION_LIMITS_UPPER ...
           | r < MOTOR_POSITION_LIMITS_LOWER ...
           | l > MOTOR_POSITION_LIMITS_UPPER ...
           | l < MOTOR_POSITION_LIMITS_LOWER);
